simulink model "SignalTracker"  (R2022a)
settings: Solver=VariableStepAuto  StartTime=0.0  StopTime=30.0  FixedStep=0.01  RelTol=1e-3
values from neighbouring files (symbols this model uses):
  toll = 1e-3    (= 0.001)    [SettingST.m]
undefined symbols (not defined in the file or in its folder): Hecate_Amp1, Hecate_Amp2, Hecate_Freq1, Hecate_Freq2, Hecate_Phase1
settings Model: Creator=The MathWorks, Inc.  LastModifiedBy=fedformi_new
settings SolverCC: AlgebraicLoopSolver=TrustRegion
settings DataIOCC: SaveFormat=Array
settings DebuggingCC: UnconnectedInputMsg=warning  UnconnectedOutputMsg=warning  UnconnectedLineMsg=warning  SFMachineParentedDataDiag=warning  ArithmeticOperatorsInVariantConditions=warning
settings SFSimCC: CustomCodeUndefinedFunction=UseInterfaceOnly

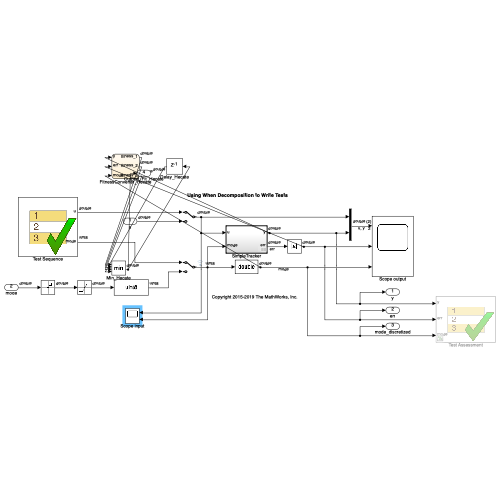
[thumbnail: Simulink's stored preview of the top-level diagram]
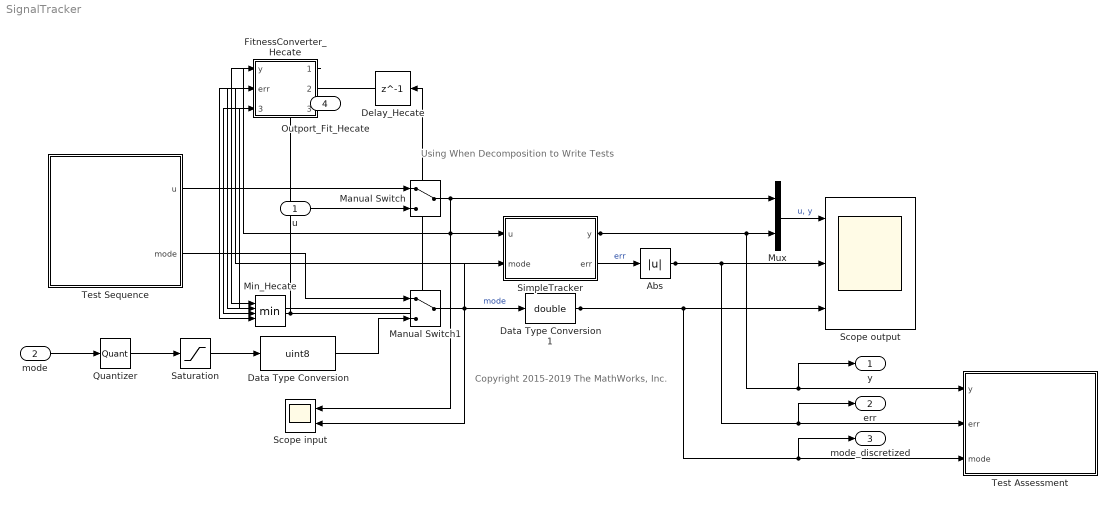
== system SignalTracker ==
  note: Using When Decomposition to Write Tests
  note: Copyright 2015-2019 The MathWorks, Inc.
  u : Inport
  mode : Inport  Port=2
  Abs : Abs  SaturateOnIntegerOverflow=off
  Data Type Conversion : DataTypeConversion  OutDataTypeStr=uint8  SaturateOnIntegerOverflow=off  RndMeth=Floor
  Data Type Conversion1 : DataTypeConversion  OutDataTypeStr=double  SaturateOnIntegerOverflow=off  RndMeth=Floor
  Delay_Hecate : Delay  DelayLength=1  InitialCondition=Inf
  FitnessConverter_Hecate : Stateflow chart  TreatAsAtomicUnit=on
  Manual Switch : ManualSwitch
  Manual Switch1 : ManualSwitch
  Min_Hecate : MinMax  Inputs=4
  Mux : Mux  Inputs=2
  Quantizer : Quantizer  QuantizationInterval=1
  Saturation : Saturate  UpperLimit=2  LowerLimit=0
  Scope input : Scope  NumInputPorts=2
  Scope output : Scope  NumInputPorts=3
  SimpleTracker : Subsystem  TreatAsAtomicUnit=on  SystemSampleTime=0.1
  Test Assessment : Test Sequence  Tag=__SLT_ASMT__  TreatAsAtomicUnit=on
  Test Sequence : Test Sequence  TreatAsAtomicUnit=on
  y : Outport
  err : Outport  Port=2
  mode_discretized : Outport  Port=3
  Outport_Fit_Hecate : Outport  Port=4
  wires:
  SimpleTracker/2(err) -> Abs/1  "err"
  Manual Switch/1 -> Mux/1, Scope input/1, SimpleTracker/1(u)
  Mux/1 -> Scope output/1  "u, y"
  Manual Switch1/1 -> Data Type Conversion1/1, SimpleTracker/2(mode), Scope input/2
  SimpleTracker/1(y) -> Mux/2, Test Assessment/1(y), y/1, FitnessConverter_Hecate/1(y)
  Test Sequence/2(mode) -> Manual Switch1/1
  Test Sequence/1(u) -> Manual Switch/1
  u/1 -> Manual Switch/2
  mode/1 -> Quantizer/1
  Quantizer/1 -> Saturation/1
  Data Type Conversion/1 -> Manual Switch1/2
  Saturation/1 -> Data Type Conversion/1
  Data Type Conversion1/1 -> Scope output/3, Test Assessment/3(mode), mode_discretized/1, FitnessConverter_Hecate/3(mode)  "mode"
  Abs/1 -> Scope output/2, err/1, Test Assessment/2(err), FitnessConverter_Hecate/2(err)
  FitnessConverter_Hecate/1(fitness_1) -> Min_Hecate/1
  FitnessConverter_Hecate/2(fitness_2) -> Min_Hecate/2
  FitnessConverter_Hecate/3(fitness_3) -> Min_Hecate/3
  Min_Hecate/1 -> Delay_Hecate/1, Outport_Fit_Hecate/1
  Delay_Hecate/1 -> Min_Hecate/4

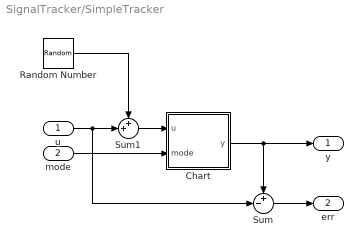
== system SignalTracker/SimpleTracker ==
  u : Inport
  mode : Inport  Port=2
  Chart : Stateflow chart  TreatAsAtomicUnit=on
  Random Number : RandomNumber  Variance=0.05  SampleTime=0.1
  Sum : Sum  Inputs=+-|
  Sum1 : Sum  Inputs=++|
  y : Outport  VectorParamsAs1DForOutWhenUnconnected=off
  err : Outport  Port=2  VectorParamsAs1DForOutWhenUnconnected=off
  wires:
  mode/1 -> Chart/2(mode)
  Chart/1(y) -> Sum/1, y/1
  u/1 -> Sum1/2, Sum/2
  Sum/1 -> err/1
  Sum1/1 -> Chart/1(u)
  Random Number/1 -> Sum1/1

== stateflow chart SignalTracker/Test Sequence ==
  state Square
    u = Hecate_Amp1 * sin(2*pi*Hecate_Freq1*et);
    state SquareAndOff
      mode = uint8(0);
    state SquareAndSlow
      mode = uint8(1);
    state SquareAndQuick
      mode = uint8(2);
    (default) -> SquareAndOff
    SquareAndOff -> SquareAndSlow : [
        | after(Hecate_Phase1, sec)
        | ]
    SquareAndSlow -> SquareAndQuick : [
        | after(Hecate_Phase1, sec)
        | ]
  state Triangle
    u = Hecate_Amp2 * triangle(Hecate_Freq2*et);
    state TriangleAndOff
      mode = uint8(0);
    state TriangleAndSlow
      mode = uint8(1);
    state TriangleAndQuick
      mode = uint8(2);
    (default) -> TriangleAndOff
    TriangleAndOff -> TriangleAndSlow : [
        | after(10-Hecate_Phase1, sec)
        | ]
    TriangleAndSlow -> TriangleAndQuick : [
        | after(10-Hecate_Phase1, sec)
        | ]
  (default) -> Square
  Square -> Triangle : [
      | after(3*Hecate_Phase1, sec)
      | ]
  data: u output double size=[1]; mode output uint8 size=[1]; Hecate_Phase1 parameter; Hecate_Amp1 parameter; Hecate_Freq1 parameter; Hecate_Amp2 parameter; Hecate_Freq2 parameter

== stateflow chart SignalTracker/FitnessConverter_Hecate ==
  state CheckError
    fitness_1 = Inf;
    fitness_2 = Inf;
    fitness_3 = Inf;
    state OffMode
      fitness_1 = Inf;
      fitness_2 = Inf;
      fitness_3 = Inf;
      state OffMode_1
        fitness_1 = Inf;
        fitness_2 = Inf;
        fitness_3 = Inf;
      state OffMode_2
        fitness_1 = toll-(abs(y));
        fitness_2 = Inf;
        fitness_3 = Inf;
      (default) -> OffMode_1
      OffMode_1 -> OffMode_2 : [et >= 0.5]
    state SlowMode
      fitness_1 = Inf;
      fitness_2 = Inf;
      fitness_3 = Inf;
      state SlowMode_1
        fitness_1 = Inf;
        fitness_2 = Inf;
        fitness_3 = Inf;
      state SlowMode_2
        fitness_1 = Inf;
        fitness_2 = 2-(err);
        fitness_3 = Inf;
      (default) -> SlowMode_1
      SlowMode_1 -> SlowMode_2 : [et >= 0.5]
    state QuickMode
      fitness_1 = Inf;
      fitness_2 = Inf;
      fitness_3 = Inf;
      state QuickMode_1
        fitness_1 = Inf;
        fitness_2 = Inf;
        fitness_3 = Inf;
      state QuickMode_2
        fitness_1 = Inf;
        fitness_2 = Inf;
        fitness_3 = 1-(err);
      (default) -> QuickMode_1
      QuickMode_1 -> QuickMode_2 : [et >= 0.5]
    state Else
      fitness_1 = Inf;
      fitness_2 = Inf;
      fitness_3 = Inf;
    Else -> (junction 4) : [(mode == 0)|(mode == 1)|(mode == 2)]
    (default) -> (junction 4)
    QuickMode -> (junction 4) : [(mode == 0)|(mode == 1)|~(mode == 2)]
    SlowMode -> (junction 4) : [(mode == 0)|~(mode == 1)]
    (junction 4) -> OffMode [order 1] : [mode == 0]
    (junction 4) -> SlowMode [order 2] : [mode == 1]
    (junction 4) -> QuickMode [order 3] : [mode == 2]
    (junction 4) -> Else [order 4] : []
    OffMode -> (junction 4) : [~(mode == 0)]
  (default) -> CheckError
  data: y input; err input; mode input; toll parameter; fitness_1 output; fitness_2 output; fitness_3 output

== stateflow chart SignalTracker/Test Assessment ==
  state Requirement
    state CheckError
      state OffMode
        state OffMode_1
        state OffMode_2
          verify(abs(y) <= toll, 'After 0.5 sec in Off, y must remain 0');
        (default) -> OffMode_1
        OffMode_1 -> OffMode_2 : [
            | et >= 0.5
            | ]
      state SlowMode
        state SlowMode_1
        state SlowMode_2
          verify(err < 2, 'After 0.5 sec in Slow, err must remain < 2');
        (default) -> SlowMode_1
        SlowMode_1 -> SlowMode_2 : [
            | et >= 0.5
            | ]
      state QuickMode
        state QuickMode_1
        state QuickMode_2
          verify(err < 1, 'After 0.5 sec in Quick, err must remain < 1');
        (default) -> QuickMode_1
        QuickMode_1 -> QuickMode_2 : [
            | et >= 0.5
            | ]
      state Else
      CheckError -> (junction 114)
      (default) -> (junction 114)
      (junction 114) -> (junction 115) [order 1] : [mode == 0
          | ]
      (junction 115) -> OffMode [order 1] : [~in(Requirement.CheckError.OffMode)]
      (junction 114) -> (junction 130) [order 2]
      (junction 115) -> (junction 118) [order 2]
      (junction 130) -> (junction 131) [order 1] : [mode == 1
          | ]
      (junction 131) -> SlowMode [order 1] : [~in(Requirement.CheckError.SlowMode)]
      (junction 130) -> (junction 145) [order 2]
      (junction 131) -> (junction 134) [order 2]
      (junction 145) -> (junction 146) [order 1] : [mode == 2
          | ]
      (junction 146) -> QuickMode [order 1] : [~in(Requirement.CheckError.QuickMode)]
      (junction 146) -> (junction 149) [order 2]
      (junction 160) -> (junction 161)
      (junction 161) -> Else [order 1] : [~in(Requirement.CheckError.Else)]
      (junction 161) -> (junction 164) [order 2]
      (junction 145) -> (junction 160) [order 2]
    (default) -> CheckError
  state Test
    state step_1
      state step_1_1
        state step_1_1_1
        state step_1_1_2
          verify(y <= toll && y >= -toll);
        (default) -> step_1_1_1
        step_1_1_1 -> step_1_1_2 : [
            | et >= 0.5
            | ]
        step_1_1_2 -> step_1_1_1 : [
            | true
            | ]
      state step_1_2
      (default) -> (junction 204)
      step_1 -> (junction 204)
      (junction 204) -> (junction 205) [order 1] : [mode <= 0.3
          | ]
      (junction 205) -> step_1_1 [order 1] : [~in(Test.step_1.step_1_1)]
      (junction 204) -> (junction 213) [order 2]
      (junction 205) -> (junction 208) [order 2]
      (junction 213) -> (junction 214)
      (junction 214) -> step_1_2 [order 1] : [~in(Test.step_1.step_1_2)]
      (junction 214) -> (junction 217) [order 2]
    (default) -> step_1
  (default) -> Requirement [order 1] : [Active_Scenario_Index == 1]
  (default) -> Test [order 2] : {assert(Active_Scenario_Index == 2,'The value of Scenario Parameter ''Active_Scenario_Index'' is not valid. Use the index of the scenario to specify it.')}
  data: y input double size=[1]; err input double size=[1]; mode input double size=[1]; toll parameter; Active_Scenario_Index parameter =1

== stateflow chart SignalTracker/SimpleTracker/Chart ==
  state TrackSlow
    en, du:
    y = y + 0.3 * (u - y);
  state TrackWait
  state TrackOff
    en:
    y = 0;
  state TrackQuick
    en, du:
    y = y + 0.7 * (u - y);
  TrackSlow -> TrackWait : [mode ~= 1]
  TrackWait -> TrackSlow [order 1] : after(0.4, sec)[mode == 1]
  TrackOff -> TrackWait : [mode ~= 0]
  (default) -> TrackOff
  TrackWait -> TrackOff [order 3] : after(0.4, sec)
  TrackQuick -> TrackWait : [mode ~= 2]
  TrackWait -> TrackQuick [order 2] : after(0.4, sec)[mode == 2]
  data: y output; u input; mode input
